simulink model "model_current"  (R2014b)
settings: Solver=ode45  StartTime=0.0  StopTime=20  RelTol=1e-3
settings Model: Creator=Annie  LastModifiedBy=Annie
settings DebuggingCC: SolverPrmCheckMsg=none

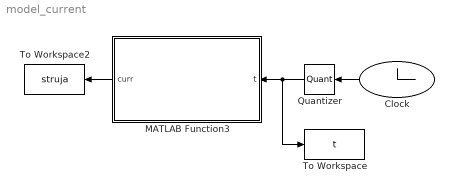
== system model_current ==
  Clock : Clock
      settings: Decimation=1000
  MATLAB Function3 : MATLAB Function  TreatAsAtomicUnit=on
  Quantizer : Quantizer  QuantizationInterval=1
  To Workspace : ToWorkspace  VariableName=t  SampleTime=-1
  To Workspace2 : ToWorkspace  VariableName=struja  SampleTime=-1
  wires:
  MATLAB Function3/1(curr) -> To Workspace2/1
  Clock/1 -> Quantizer/1
  Quantizer/1 -> To Workspace/1, MATLAB Function3/1(t)

== matlab function model_current/MATLAB Function3 ==
  data: curr output; t input
function curr = current (t)
%#codegen

alfa_rad =0;
v_x=0;
v_y=0;
v = 0;

persistent brojac;
if isempty(brojac)
    brojac = 0;
end

persistent alfa;
if isempty(alfa)
    alfa = 0;
end


if t<20
    
    if mod(t, 3) == 0 & floor(t/3) > brojac
        
        brojac = brojac +1;
        alfa = alfa+3;
        
        if mod(alfa, 360) == 0
            alfa=0
        end    
    end
end

alfa_rad = alfa * pi / 180;
v=1;
v_x= v * sin(alfa_rad);
v_y= v * cos(alfa_rad);

curr=[v_x v_y];
        
end
